simulink subsystem "Twist_Publisher"  (R2022b)
settings: Solver=VariableStepAuto  StartTime=0.0  StopTime=10.0  RelTol=1e-3
undefined symbols (not defined in the file): header, twist
libraries: ros2lib x2, simulink_extras x1
settings Model: Creator=hayden  LastModifiedBy=hollis
settings ModelReferenceCC: EnableRefExpFcnMdlSchedulingChecks=on

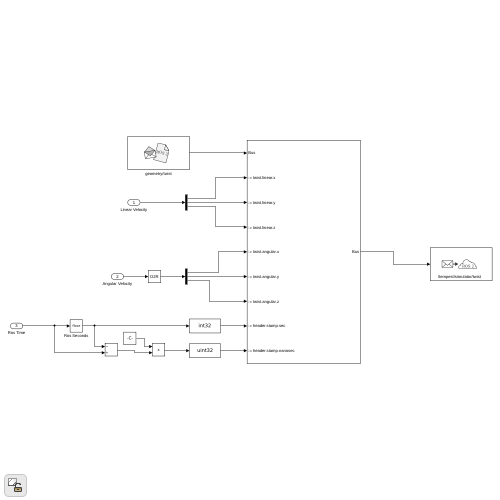
[thumbnail: Simulink's stored preview of the top-level diagram]
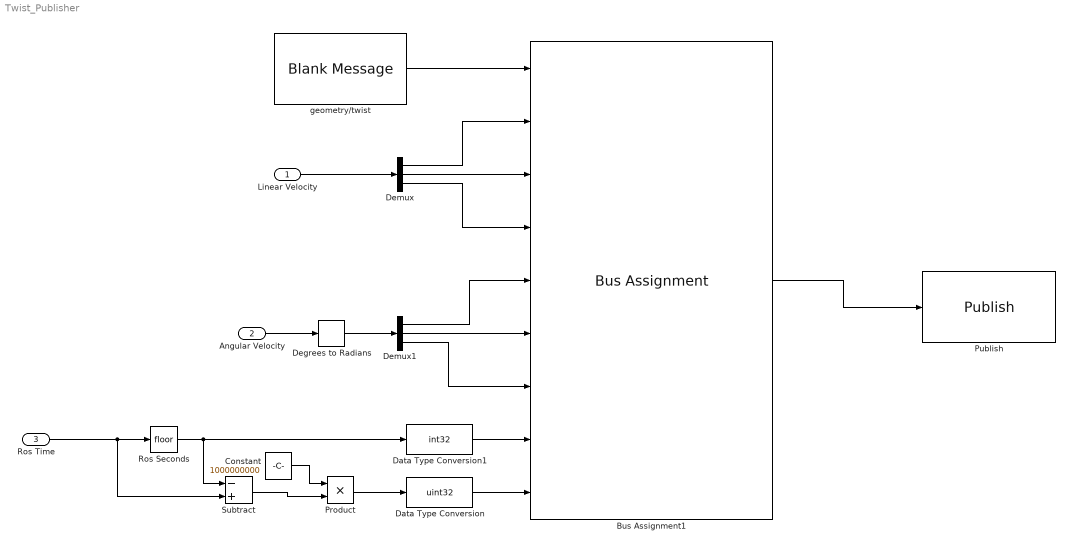
== system Twist_Publisher ==
  Linear Velocity : Inport
  Angular Velocity : Inport  Port=2
  Ros Time : Inport  Port=3
  Bus Assignment1 : BusAssignment  AssignedSignals=twist.linear.x,twist.linear.y,twist.linear.z,twist.angular.x,twist.angular.y,twist.angular.z,header.stamp.sec,header.stamp.nanosec
  Constant : Constant  Value=1000000000
  Data Type Conversion : DataTypeConversion  OutDataTypeStr=uint32  SaturateOnIntegerOverflow=off  RndMeth=Floor
  Data Type Conversion1 : DataTypeConversion  OutDataTypeStr=int32  SaturateOnIntegerOverflow=off  RndMeth=Floor
  Degrees to Radians : simulink_extras/Transformations/Degrees to Radians
  Demux : Demux  Outputs=3
  Demux1 : Demux  Outputs=3
  Product : Product
  Publish : ros2lib/Publish  topicSource=Select from ROS network  topic=/talos/simulator/twist  messageType=geometry_msgs/TwistStamped  QOSHistory=Keep last  QOSDepth=1  QOSReliability=Reliable  QOSDurability=Volatile
  Ros Seconds : Rounding
  Subtract : Sum  Inputs=-+
  geometry/twist : ros2lib/Blank Message  messageClass=Message  entityType=geometry_msgs/TwistStamped  messageType=geometry_msgs/TwistStamped  SampleTime=inf
  wires:
  geometry/twist/1 -> Bus Assignment1/1
  Bus Assignment1/1 -> Publish/1
  Demux/2 -> Bus Assignment1/3
  Demux/1 -> Bus Assignment1/2
  Demux/3 -> Bus Assignment1/4
  Demux1/2 -> Bus Assignment1/6
  Demux1/1 -> Bus Assignment1/5
  Demux1/3 -> Bus Assignment1/7
  Linear Velocity/1 -> Demux/1
  Angular Velocity/1 -> Degrees to Radians/1
  Ros Seconds/1 -> Subtract/1, Data Type Conversion1/1
  Constant/1 -> Product/1
  Subtract/1 -> Product/2
  Ros Time/1 -> Ros Seconds/1, Subtract/2
  Product/1 -> Data Type Conversion/1
  Data Type Conversion/1 -> Bus Assignment1/9
  Data Type Conversion1/1 -> Bus Assignment1/8
  Degrees to Radians/1 -> Demux1/1
